simulink model "BiPAP_Architecture"  (R2022b)
settings: Solver=VariableStepAuto  StartTime=0.0  StopTime=10.0  RelTol=1e-3
settings Model: Creator=Wayne  LastModifiedBy=MATLAB
settings DebuggingCC: UnconnectedInputMsg=warning  UnconnectedOutputMsg=warning  UnconnectedLineMsg=warning
settings ModelReferenceCC: EnableRefExpFcnMdlSchedulingChecks=on
settings RTWCC: DLArmComputeVersion=19.05

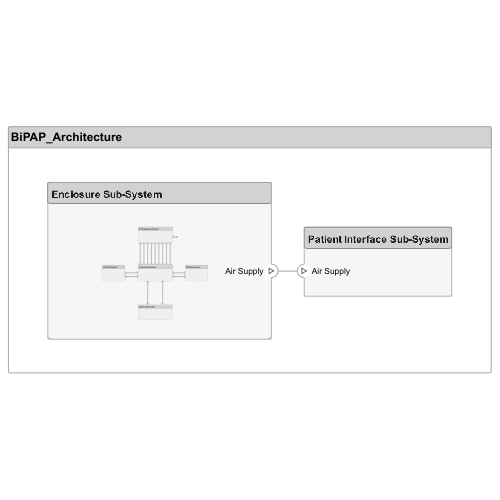
[thumbnail: Simulink's stored preview of the top-level diagram]
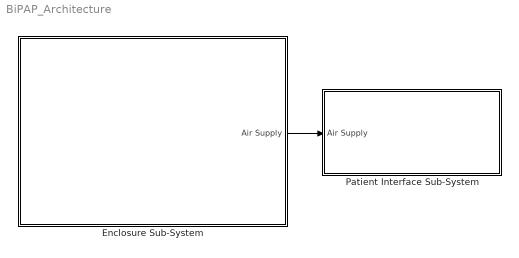
== system BiPAP_Architecture ==
  Enclosure Sub-System : Subsystem
      settings: PortSchema="{\"entries\":[{\"content\":{\"headerSize\":26,\"margin\":15,\"minimumSpacing\":25,\"sides\":[{\"content\":{\"connectorIds\":[]},\"type\":\"ConnectorPlacement.EquallySpacedRectSide\",\"uuid\":\"81d5b4bf-3469-4477-be1d-3733ca69d7c0\"},{\"content\":{\"connectorIds\":[\"Out1\"],\"side\":\"RIGHT\"},\"type\":\"ConnectorPlacement.EquallySpacedRectSide\",\"uuid\":\"66441187-0c8a-4507-bd97-68d2700f7568\"},{\"content\":{\"connectorIds\":[],\"side\":\"TOP\"},\"type\":\"ConnectorPlacement.EquallySpacedRectSide\",\"uuid\":\"afd044d7-1d3c-4759-b7a3-84d9a7d3570f\"},{\"content\":{\"connectorIds\":[],\"side\":\"HIDDEN\"},\"type\":\"ConnectorPlacement.EquallySpacedRectSide\",\"uuid\":\"77362e5b-0622-439c-804c-be4eee9d3d34\"}]},\"type\":\"ConnectorPlacement.EquallySpacedConnector\",\"uuid\":\"62deff30-9026-411d-9cb6-6c4e111723da\"}],\"packageUris\":[\"http://schema.mathworks.com/mf0/Connector/R2020b\"],\"version\":\"1.0\"}"
  Patient Interface Sub-System : Subsystem
      settings: PortSchema="{\"entries\":[{\"content\":{\"headerSize\":26,\"margin\":15,\"minimumSpacing\":25,\"sides\":[{\"content\":{\"connectorIds\":[\"In1\"]},\"type\":\"ConnectorPlacement.EquallySpacedRectSide\",\"uuid\":\"81d5b4bf-3469-4477-be1d-3733ca69d7c0\"},{\"content\":{\"connectorIds\":[],\"side\":\"RIGHT\"},\"type\":\"ConnectorPlacement.EquallySpacedRectSide\",\"uuid\":\"66441187-0c8a-4507-bd97-68d2700f7568\"},{\"content\":{\"connectorIds\":[],\"side\":\"TOP\"},\"type\":\"ConnectorPlacement.EquallySpacedRectSide\",\"uuid\":\"afd044d7-1d3c-4759-b7a3-84d9a7d3570f\"},{\"content\":{\"connectorIds\":[],\"side\":\"HIDDEN\"},\"type\":\"ConnectorPlacement.EquallySpacedRectSide\",\"uuid\":\"77362e5b-0622-439c-804c-be4eee9d3d34\"}]},\"type\":\"ConnectorPlacement.EquallySpacedConnector\",\"uuid\":\"62deff30-9026-411d-9cb6-6c4e111723da\"}],\"packageUris\":[\"http://schema.mathworks.com/mf0/Connector/R2020b\"],\"version\":\"1.0\"}"
  wires:
  Enclosure Sub-System/1(Air Supply) -> Patient Interface Sub-System/1(Air Supply)

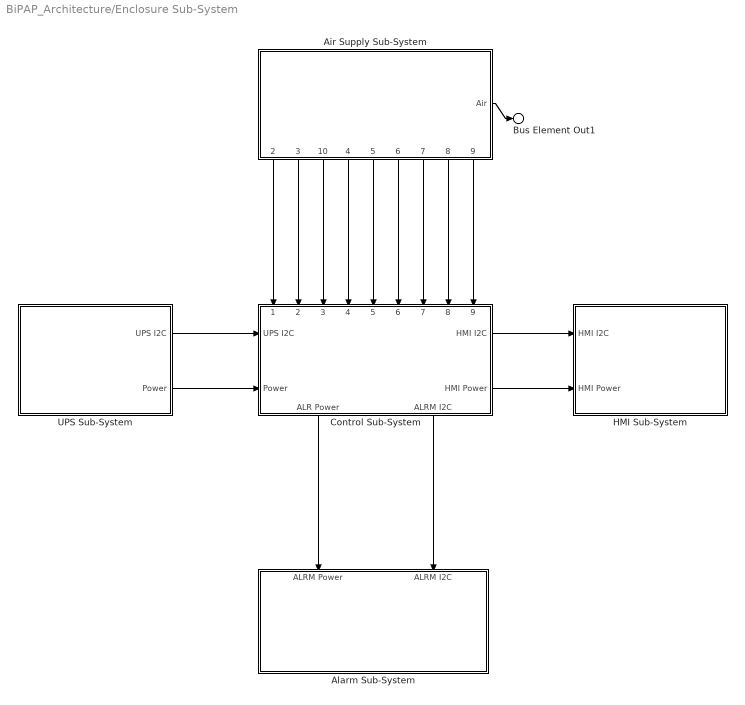
== system BiPAP_Architecture/Enclosure Sub-System ==
  Air Supply Sub-System : Subsystem
      settings: PortSchema="{\"entries\":[{\"content\":{\"headerSize\":26,\"margin\":15,\"minimumSpacing\":25,\"sides\":[{\"content\":{\"connectorIds\":[]},\"type\":\"ConnectorPlacement.EquallySpacedRectSide\",\"uuid\":\"81d5b4bf-3469-4477-be1d-3733ca69d7c0\"},{\"content\":{\"connectorIds\":[\"Out1\"],\"side\":\"RIGHT\"},\"type\":\"ConnectorPlacement.EquallySpacedRectSide\",\"uuid\":\"66441187-0c8a-4507-bd97-68d2700f7568\"},{\"content\":{\"connectorIds\":[],\"side\":\"TOP\"},\"type\":\"ConnectorPlacement.EquallySpacedRectSide\",\"uuid\":\"afd044d7-1d3c-4759-b7a3-84d9a7d3570f\"},{\"content\":{\"connectorIds\":[\"Out2\",\"Out3\",\"Out10\",\"Out4\",\"Out5\",\"Out6\",\"Out7\",\"Out8\",\"Out9\"],\"side\":\"BOTTOM\"},\"type\":\"ConnectorPlacement.EquallySpacedRectSide\",\"uuid\":\"c617ac4b-28a0-4f76-be59-d4ffba132025\"},{\"content\":{\"connectorIds\":[],\"side\":\"HIDDEN\"},\"type\":\"ConnectorPlacement.EquallySpacedRectSide\",\"uuid\":\"77362e5b-0622-439c-804c-be4eee9d3d34\"}]},\"type\":\"ConnectorPlacement.EquallySpacedConnector\",\"uuid\":\"62deff30-9026-411d-9cb6-6c4e111723da\"}],\"packageUris\":[\"http://schema.mathworks.com/mf0/Connector/R2020b\"],\"version\":\"1.0\"}"
  Alarm Sub-System : Subsystem
      settings: PortSchema="{\"entries\":[{\"content\":{\"headerSize\":26,\"margin\":15,\"minimumSpacing\":25,\"sides\":[{\"content\":{\"connectorIds\":[]},\"type\":\"ConnectorPlacement.EquallySpacedRectSide\",\"uuid\":\"81d5b4bf-3469-4477-be1d-3733ca69d7c0\"},{\"content\":{\"connectorIds\":[],\"side\":\"RIGHT\"},\"type\":\"ConnectorPlacement.EquallySpacedRectSide\",\"uuid\":\"66441187-0c8a-4507-bd97-68d2700f7568\"},{\"content\":{\"connectorIds\":[\"In1\",\"In2\"],\"side\":\"TOP\"},\"type\":\"ConnectorPlacement.EquallySpacedRectSide\",\"uuid\":\"afd044d7-1d3c-4759-b7a3-84d9a7d3570f\"},{\"content\":{\"connectorIds\":[],\"side\":\"HIDDEN\"},\"type\":\"ConnectorPlacement.EquallySpacedRectSide\",\"uuid\":\"77362e5b-0622-439c-804c-be4eee9d3d34\"}]},\"type\":\"ConnectorPlacement.EquallySpacedConnector\",\"uuid\":\"62deff30-9026-411d-9cb6-6c4e111723da\"}],\"packageUris\":[\"http://schema.mathworks.com/mf0/Connector/R2020b\"],\"version\":\"1.0\"}"
  Control Sub-System : Subsystem
      settings: PortSchema="{\"entries\":[{\"content\":{\"headerSize\":26,\"margin\":15,\"minimumSpacing\":25,\"sides\":[{\"content\":{\"connectorIds\":[\"In10\",\"In11\"]},\"type\":\"ConnectorPlacement.EquallySpacedRectSide\",\"uuid\":\"81d5b4bf-3469-4477-be1d-3733ca69d7c0\"},{\"content\":{\"connectorIds\":[\"Out1\",\"Out2\"],\"side\":\"RIGHT\"},\"type\":\"ConnectorPlacement.EquallySpacedRectSide\",\"uuid\":\"66441187-0c8a-4507-bd97-68d2700f7568\"},{\"content\":{\"connectorIds\":[\"In1\",\"In2\",\"In3\",\"In4\",\"In5\",\"In6\",\"In7\",\"In8\",\"In9\"],\"side\":\"TOP\"},\"type\":\"ConnectorPlacement.EquallySpacedRectSide\",\"uuid\":\"afd044d7-1d3c-4759-b7a3-84d9a7d3570f\"},{\"content\":{\"connectorIds\":[\"Out3\",\"Out4\"],\"side\":\"BOTTOM\"},\"type\":\"ConnectorPlacement.EquallySpacedRectSide\",\"uuid\":\"1822936f-0510-4202-b591-b78152b78dc4\"},{\"content\":{\"connectorIds\":[],\"side\":\"HIDDEN\"},\"type\":\"ConnectorPlacement.EquallySpacedRectSide\",\"uuid\":\"77362e5b-0622-439c-804c-be4eee9d3d34\"}]},\"type\":\"ConnectorPlacement.EquallySpacedConnector\",\"uuid\":\"62deff30-9026-411d-9cb6-6c4e111723da\"}],\"packageUris\":[\"http://schema.mathworks.com/mf0/Connector/R2020b\"],\"version\":\"1.0\"}"
  HMI Sub-System : Subsystem
      settings: PortSchema="{\"entries\":[{\"content\":{\"headerSize\":26,\"margin\":15,\"minimumSpacing\":25,\"sides\":[{\"content\":{\"connectorIds\":[\"In1\",\"In2\"]},\"type\":\"ConnectorPlacement.EquallySpacedRectSide\",\"uuid\":\"81d5b4bf-3469-4477-be1d-3733ca69d7c0\"},{\"content\":{\"connectorIds\":[],\"side\":\"RIGHT\"},\"type\":\"ConnectorPlacement.EquallySpacedRectSide\",\"uuid\":\"66441187-0c8a-4507-bd97-68d2700f7568\"},{\"content\":{\"connectorIds\":[],\"side\":\"TOP\"},\"type\":\"ConnectorPlacement.EquallySpacedRectSide\",\"uuid\":\"afd044d7-1d3c-4759-b7a3-84d9a7d3570f\"},{\"content\":{\"connectorIds\":[],\"side\":\"HIDDEN\"},\"type\":\"ConnectorPlacement.EquallySpacedRectSide\",\"uuid\":\"77362e5b-0622-439c-804c-be4eee9d3d34\"}]},\"type\":\"ConnectorPlacement.EquallySpacedConnector\",\"uuid\":\"62deff30-9026-411d-9cb6-6c4e111723da\"}],\"packageUris\":[\"http://schema.mathworks.com/mf0/Connector/R2020b\"],\"version\":\"1.0\"}"
  UPS Sub-System : Subsystem
      settings: PortSchema="{\"entries\":[{\"content\":{\"headerSize\":26,\"margin\":15,\"minimumSpacing\":25,\"sides\":[{\"content\":{\"connectorIds\":[]},\"type\":\"ConnectorPlacement.EquallySpacedRectSide\",\"uuid\":\"81d5b4bf-3469-4477-be1d-3733ca69d7c0\"},{\"content\":{\"connectorIds\":[\"Out1\",\"Out2\"],\"side\":\"RIGHT\"},\"type\":\"ConnectorPlacement.EquallySpacedRectSide\",\"uuid\":\"66441187-0c8a-4507-bd97-68d2700f7568\"},{\"content\":{\"connectorIds\":[],\"side\":\"TOP\"},\"type\":\"ConnectorPlacement.EquallySpacedRectSide\",\"uuid\":\"afd044d7-1d3c-4759-b7a3-84d9a7d3570f\"},{\"content\":{\"connectorIds\":[],\"side\":\"HIDDEN\"},\"type\":\"ConnectorPlacement.EquallySpacedRectSide\",\"uuid\":\"77362e5b-0622-439c-804c-be4eee9d3d34\"}]},\"type\":\"ConnectorPlacement.EquallySpacedConnector\",\"uuid\":\"62deff30-9026-411d-9cb6-6c4e111723da\"}],\"packageUris\":[\"http://schema.mathworks.com/mf0/Connector/R2020b\"],\"version\":\"1.0\"}"
  Bus Element Out1 : Outport  PortName=Air Supply
  wires:
  Air Supply Sub-System/4(CAN Bus) -> Control Sub-System/4(CAN Bus)
  Control Sub-System/3(ALR Power) -> Alarm Sub-System/1(ALRM Power)
  Control Sub-System/1(HMI I2C) -> HMI Sub-System/1(HMI I2C)
  Control Sub-System/4(ALRM I2C) -> Alarm Sub-System/2(ALRM I2C)
  UPS Sub-System/1(UPS I2C) -> Control Sub-System/10(UPS I2C)
  Air Supply Sub-System/9(Motor Brake) -> Control Sub-System/9(Motor Brake)
  UPS Sub-System/2(Power) -> Control Sub-System/11(Power)
  Air Supply Sub-System/3(AS I2C_1) -> Control Sub-System/2(AS I2C_1)
  Air Supply Sub-System/2(AS Power) -> Control Sub-System/1(AS Power)
  Air Supply Sub-System/10(AS I2C_2) -> Control Sub-System/3(AS I2C_2)
  Control Sub-System/2(HMI Power) -> HMI Sub-System/2(HMI Power)
  Air Supply Sub-System/1(Air) -> Bus Element Out1/1
  Air Supply Sub-System/8(Motor Disable) -> Control Sub-System/8(Motor Disable)
  Air Supply Sub-System/7(Motor Speed) -> Control Sub-System/7(Motor Speed)
  Air Supply Sub-System/5(Anologue_1) -> Control Sub-System/5(Anologue_1)
  Air Supply Sub-System/6(Anologue_2) -> Control Sub-System/6(Anologue_2)

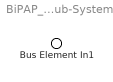
== system BiPAP_Architecture/Patient Interface Sub-System ==
  Bus Element In1 : Inport  PortName=Air Supply

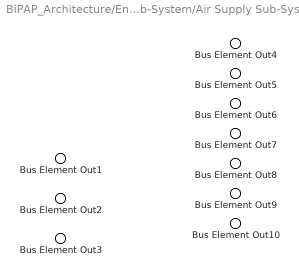
== system BiPAP_Architecture/Enclosure Sub-System/Air Supply Sub-System ==
  Bus Element Out4 : Outport  PortName=Air
  Bus Element Out1 : Outport  Port=2  PortName=AS Power
  Bus Element Out2 : Outport  Port=3  PortName=AS I2C_1
  Bus Element Out5 : Outport  Port=4  PortName=CAN Bus
  Bus Element Out6 : Outport  Port=5  PortName=Anologue_1
  Bus Element Out7 : Outport  Port=6  PortName=Anologue_2
  Bus Element Out8 : Outport  Port=7  PortName=Motor Speed
  Bus Element Out9 : Outport  Port=8  PortName=Motor Disable
  Bus Element Out10 : Outport  Port=9  PortName=Motor Brake
  Bus Element Out3 : Outport  Port=10  PortName=AS I2C_2

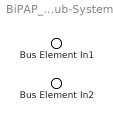
== system BiPAP_Architecture/Enclosure Sub-System/Alarm Sub-System ==
  Bus Element In1 : Inport  PortName=ALRM Power
  Bus Element In2 : Inport  Port=2  PortName=ALRM I2C

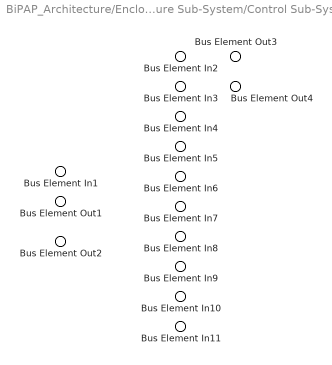
== system BiPAP_Architecture/Enclosure Sub-System/Control Sub-System ==
  Bus Element In3 : Inport  PortName=AS Power
  Bus Element In4 : Inport  Port=2  PortName=AS I2C_1
  Bus Element In5 : Inport  Port=3  PortName=AS I2C_2
  Bus Element In6 : Inport  Port=4  PortName=CAN Bus
  Bus Element In7 : Inport  Port=5  PortName=Anologue_1
  Bus Element In8 : Inport  Port=6  PortName=Anologue_2
  Bus Element In9 : Inport  Port=7  PortName=Motor Speed
  Bus Element In10 : Inport  Port=8  PortName=Motor Disable
  Bus Element In11 : Inport  Port=9  PortName=Motor Brake
  Bus Element In2 : Inport  Port=10  PortName=UPS I2C
  Bus Element In1 : Inport  Port=11  PortName=Power
  Bus Element Out4 : Outport  PortName=HMI I2C
  Bus Element Out3 : Outport  Port=2  PortName=HMI Power
  Bus Element Out1 : Outport  Port=3  PortName=ALR Power
  Bus Element Out2 : Outport  Port=4  PortName=ALRM I2C

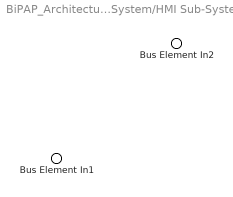
== system BiPAP_Architecture/Enclosure Sub-System/HMI Sub-System ==
  Bus Element In2 : Inport  PortName=HMI I2C
  Bus Element In1 : Inport  Port=2  PortName=HMI Power

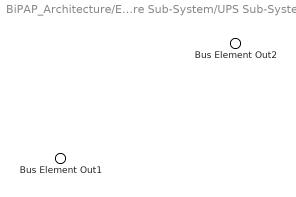
== system BiPAP_Architecture/Enclosure Sub-System/UPS Sub-System ==
  Bus Element Out2 : Outport  PortName=UPS I2C
  Bus Element Out1 : Outport  Port=2  PortName=Power
